simulink model "controlForThermo_simulink"  (R2022a)
settings: Solver=VariableStepAuto  StartTime=0.0  StopTime=10.0  RelTol=1e-3
settings Model: Creator=Anupp  LastModifiedBy=Anupp

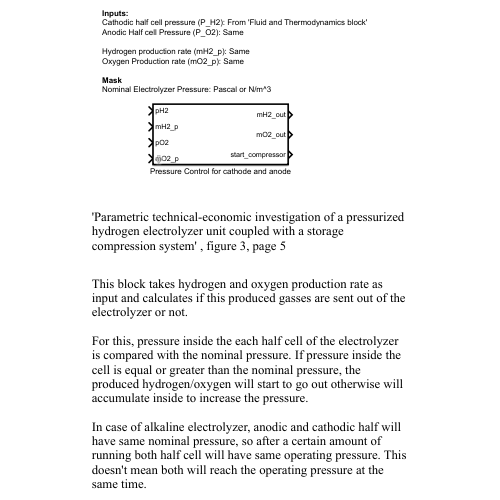
[thumbnail: Simulink's stored preview of the top-level diagram]
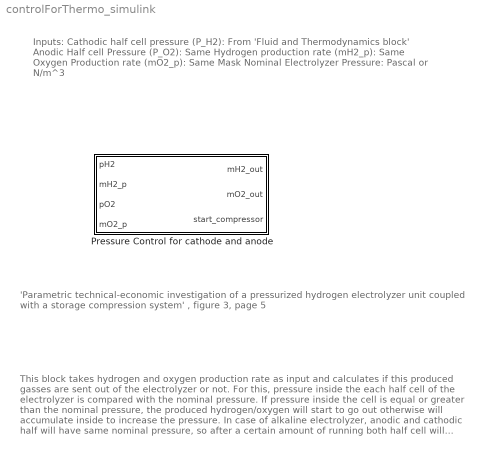
== system controlForThermo_simulink ==
  note: Inputs:
      | Cathodic half cell pressure (P_H2): From 'Fluid and Thermodynamics block'
      | Anodic Half cell Pressure (P_O2): Same
      |
      | Hydrogen production rate (mH2_p): Same
      | Oxygen Production rate (mO2_p): Same
      |
      | Mask
      | Nominal Electrolyzer Pressure: Pascal or N/m^3
  note: 'Parametric technical-economic investigation of a pressurized hydrogen electrolyzer unit coupled with a storage compression system' , figure 3, page 5
  note: This block takes hydrogen and oxygen production rate as input and calculates if this produced gasses are sent out of the electrolyzer or not.
      |
      | For this, pressure inside the each half cell of the electrolyzer is compared with the nominal pressure. If pressure inside the cell is equal or greater than the nominal pressure, the produced hydrogen/oxygen will start to go out otherwise will accumulate inside to increase the pressure.
      |
      | In case of alkaline electrolyzer, anodic and cathodic half will have same nominal pressure, so after a certain amount of running both half cell will have same operating pressure. This doesn't mean both will reach the operating pressure at the same time.
  Pressure Control for cathode and anode : Subsystem  TreatAsAtomicUnit=on  mask{P_nominal=0}
      mask prompts: P_nominal "Nominal Electrolyzer Pressure"

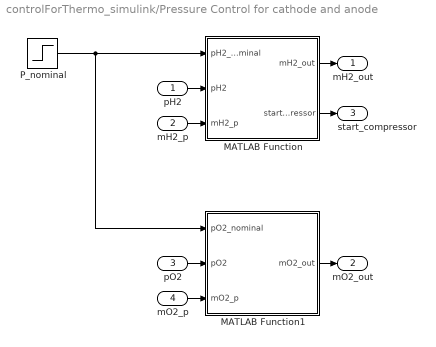
== system controlForThermo_simulink/Pressure Control for cathode and anode ==
  pH2 : Inport
  mH2_p : Inport  Port=2
  pO2 : Inport  Port=3
  mO2_p : Inport  Port=4
  MATLAB Function : MATLAB Function  TreatAsAtomicUnit=on
  MATLAB Function1 : MATLAB Function  TreatAsAtomicUnit=on
  P_nominal : Step  Time=0  After=P_nominal  SampleTime=0
  mH2_out : Outport
  mO2_out : Outport  Port=2
  start_compressor : Outport  Port=3
  wires:
  P_nominal/1 -> MATLAB Function1/1(pO2_nominal), MATLAB Function/1(pH2_nominal)
  mH2_p/1 -> MATLAB Function/3(mH2_p)
  MATLAB Function/2(start_compressor) -> start_compressor/1
  MATLAB Function/1(mH2_out) -> mH2_out/1
  pH2/1 -> MATLAB Function/2(pH2)
  MATLAB Function1/1(mO2_out) -> mO2_out/1
  mO2_p/1 -> MATLAB Function1/3(mO2_p)
  pO2/1 -> MATLAB Function1/2(pO2)

== matlab function controlForThermo_simulink/Pressure Control for cathode and anode/MATLAB Function1 ==
  data: pO2_nominal input; mO2_out output; pO2 input; mO2_p input
%% Inputs:
% mass of Oxygen prod. : kg/s
% pressure at anode : Pascal or N/m^3
% nominal pressure : pascal or N/m^3

%% Outputs:
% Oxygen mass out: Kg/s
% start compressor signal : 1 or 0

% If pressure at anode is greater than or equal to nominal pressure
% compressor is started and all produced Oxygen is sent out

% If pressure at anode is less than nominal pressure
% produced Oxygen is let to accumulate, H2_out is set 0

% '1' is used as compressor on and '0' as off

%% Main Function



function mO2_out  = fcn(pO2_nominal,pO2,mO2_p)

    if pO2 >= pO2_nominal
        mO2_out = mO2_p;
    else
        mO2_out = 0;
    end
end

== matlab function controlForThermo_simulink/Pressure Control for cathode and anode/MATLAB Function ==
  data: pH2_nominal input; mH2_out output; pH2 input; mH2_p input; start_compressor output
%% Inputs:
% mass of hydrogen prod. : kg/s
% pressure at cathode : Pascal or N/m^3
% nominal pressure : pascal or N/m^3

%% Outputs:
% Hydrogen mass out: Kg/s
% start compressor signal : 1 or 0

% If pressure at cathode is greater than or equal to nominal pressure
% compressor is started and all produced hydrogen is sent out

% If pressure at cathode is less than nominal pressure
% produced hydrogen is let to accumulate, H2_out is set 0

% '1' is used as compressor on and '0' as off

%% Main Function

function [mH2_out,start_compressor]  = fcn(pH2_nominal,pH2,mH2_p)

    if pH2 >= pH2_nominal
        mH2_out = mH2_p;
        start_compressor = 1;
    else
        mH2_out = 0;
        start_compressor = 0;
    end
end
